simulink model "Elektromagnet_MV_V10_erweitert"  (R2016a)
settings: Solver=ode45  StartTime=0.0  StopTime=0.5  FixedStep=0.001  RelTol=1e-3
values from neighbouring files (symbols this model uses):
  A = 37.7*0.000001    (= 3.77e-05)    [Skript_Elektromagnet_MV_V10_erweitert.m]
  A_v = 0.002^2*pi()/4    [Skript_Elektromagnet_MV_V10_erweitert.m]
  c_Feder = 1000    [Skript_Elektromagnet_MV_V10_erweitert.m]
  d_Daempfer = 10    [Skript_Elektromagnet_MV_V10_erweitert.m]
  F_vorspann = 0.5    [Skript_Elektromagnet_MV_V10_erweitert.m]
  lges = 0.06    [Skript_Elektromagnet_MV_V10_erweitert.m]
  m = 0.010    (= 0.01)    [Skript_Elektromagnet_MV_V10_erweitert.m]
  maxhub = 0.002    [Skript_Elektromagnet_MV_V10_erweitert.m]
  my0 = 1.257*0.000001    (= 1.257e-06)    [Skript_Elektromagnet_MV_V10_erweitert.m]
  myr = 50    [Skript_Elektromagnet_MV_V10_erweitert.m]
  p = pVec(i)    [Skript_Elektromagnet_MV_V10_erweitert.m]
  R = 11    [Skript_Elektromagnet_MV_V10_erweitert.m]
  Ui = p    [Skript_Elektromagnet_MV_V10_erweitert.m]
  w = 800    [Skript_Elektromagnet_MV_V10_erweitert.m]
settings Model: Creator=niebergall  LastModifiedBy=Michaél
settings DataIOCC: LimitDataPoints=on  SaveFormat=Array
settings DebuggingCC: UnderspecifiedInitializationDetection=Classic  MergeDetectMultiDrivingBlocksExec=none  StateNameClashWarn=warning
settings HardwareCC: ProdBitPerPointer=32  ProdLargestAtomicFloat=None  ProdIntDivRoundTo=Undefined  ProdEndianess=Unspecified  ProdWordSize=32  ProdHWDeviceType=32-bit Generic
settings ModelReferenceCC: PropagateSignalLabelsOutOfModel=off
settings ConfigComp: CovModelRefEnable=Off

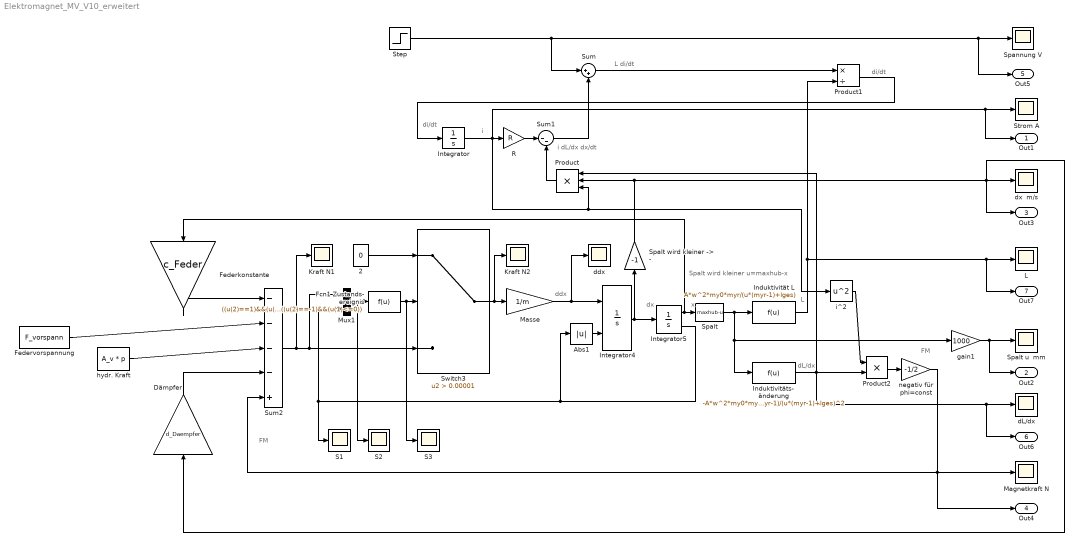
== system Elektromagnet_MV_V10_erweitert ==
  note: Spalt wird kleiner
      | u=maxhub-x
  note: di/dt
  note: FM
  note: FM
  note: dL/dx
  note: L
  note: i dL/dx dx/dt
  note: di/dt
  note: i
  note: L di/dt
  note: x
  note: dx
  note: ddx
  2 : Constant  Value=0
  Abs1 : Abs
  Dämpfer : Gain  Gain=d_Daempfer
  Fcn1 Zustands- ereignis : Fcn  Expr=((u(2)==1)&&(u(1)>=0)) || ((u(2)==-1)&&(u(1)<=0))
  Federkonstante : Gain  Gain=c_Feder
  Federvorspannung : Constant  Value=F_vorspann
  Induktivität L : Fcn  Expr=A*w^2*my0*myr/(u*(myr-1)+lges)
  Induktivitäts- änderung : Fcn  Expr=-A*w^2*my0*myr*(myr-1)/(u*(myr-1)+lges)^2
  Integrator : Integrator
  Integrator4 : Integrator  ExternalReset=rising
  Integrator5 : Integrator  LimitOutput=on  UpperSaturationLimit=maxhub  LowerSaturationLimit=0  ShowSaturationPort=on
  Kraft N1 : Scope
  Kraft N2 : Scope
  L : Scope
  Magnetkraft N : Scope
  Masse : Gain  Gain=1/m
  Mux1 : Mux  Inputs=2
  Product : Product  Inputs=3
  Product1 : Product  Inputs=*/
  Product2 : Product
  R : Gain  Gain=R
  S1 : Scope
  S2 : Scope
  S3 : Scope
  Spalt : Fcn  Expr=maxhub-u
  Spalt u  mm : Scope
  "Spalt wird kleiner -> -" : Gain  Gain=-1
  Spannung V : Scope
  Step : Step  Time=0  After=Ui  SampleTime=0
  Strom A : Scope
  Sum : Sum  Inputs=|++
  Sum1 : Sum  Inputs=|--
  Sum2 : Sum  Inputs=|----+
  Switch3 : Switch  Criteria=u2 > Threshold  Threshold=0.00001
  dL/dx : Scope
  ddx : Scope
  dx  m/s : Scope
  gain1 : Gain  Gain=1000
  hydr. Kraft : Constant  Value=A_v * p
  i^2 : Math  Operator=square  SaturateOnIntegerOverflow=on
  negativ für phi=const : Gain  Gain=-1/2
  Out1 : Outport
  Out2 : Outport  Port=2
  Out3 : Outport  Port=3
  Out4 : Outport  Port=4
  Out5 : Outport  Port=5
  Out6 : Outport  Port=6
  Out7 : Outport  Port=7
  wires:
  Sum/1 -> Product1/1
  R/1 -> Sum1/1
  Sum1/1 -> Sum/2
  Product/1 -> Sum1/2
  Induktivitäts- änderung/1 -> Product/1, Product2/2, Out6/1, dL/dx/1
  i^2/1 -> Product2/1
  Product2/1 -> negativ für phi=const/1
  Product1/1 -> Integrator/1
  Integrator/1 -> Product/3, i^2/1, Out1/1, Strom A/1, R/1
  Step/1 -> Sum/1, Out5/1, Spannung V/1
  Induktivität L/1 -> Product1/2, Out7/1, L/1
  negativ für phi=const/1 -> Sum2/5, Out4/1, Magnetkraft N/1
  2/1 -> Switch3/1
  Fcn1 Zustands- ereignis/1 -> S3/1, Switch3/2
  Mux1/1 -> S2/1, Fcn1 Zustands- ereignis/1
  Sum2/1 -> Kraft N1/1, Switch3/3, Mux1/1
  Integrator4/1 -> Integrator5/1, "Spalt wird kleiner -> -"/1
  Abs1/1 -> Integrator4/2
  Masse/1 -> Integrator4/1, ddx/1
  Switch3/1 -> Masse/1, Kraft N2/1
  Integrator5/2 -> S1/1, Mux1/2, Abs1/1
  Spalt/1 -> Induktivitäts- änderung/1, gain1/1, Induktivität L/1
  "Spalt wird kleiner -> -"/1 -> dx  m/s/1, Dämpfer/1, Out3/1, Product/2
  Federkonstante/1 -> Sum2/1
  Dämpfer/1 -> Sum2/4
  gain1/1 -> Out2/1, Spalt u  mm/1
  Federvorspannung/1 -> Sum2/2
  Integrator5/1 -> Federkonstante/1, Spalt/1
  hydr. Kraft/1 -> Sum2/3
